simulink model "track5p"  (Simulink 9.0)
settings: Solver=ode1  StartTime=0.0  StopTime=120  RelTol=1e-3
libraries: simulink x2, Solver_SF x1
settings Model: Creator=lancer  LastModifiedBy=lancer
settings DataIOCC: SaveFormat=Dataset
settings OptimizationCC: LifeSpan=auto
settings DebuggingCC: UnderspecifiedInitializationDetection=Simplified  MergeDetectMultiDrivingBlocksExec=error  SFUnexpectedBacktrackingDiag=error  SFNoUnconditionalDefaultTransitionDiag=error  SFExecutionAtInitializationDiag=warning
settings HardwareCC: ProdBitPerPointer=64  ProdBitPerSizeT=64  ProdBitPerPtrDiffT=64  ProdLargestAtomicFloat=Float  ProdIntDivRoundTo=Zero  ProdEndianess=LittleEndian  ProdWordSize=64  ProdHWDeviceType=Intel->x86-64 (Windows64)
settings ModelReferenceCC: PropagateSignalLabelsOutOfModel=on
settings CodeAppCC: StateflowObjectComments=off
settings GRTTargetCC: TargetLangStandard=C99 (ISO)
settings ConfigComp: CovMetricSettings=dwe  CovHtmlReporting=off  CovSaveCumulativeToWorkspaceVar=off  CovSaveSingleToWorkspaceVar=off  CovExternalEMLEnable=on

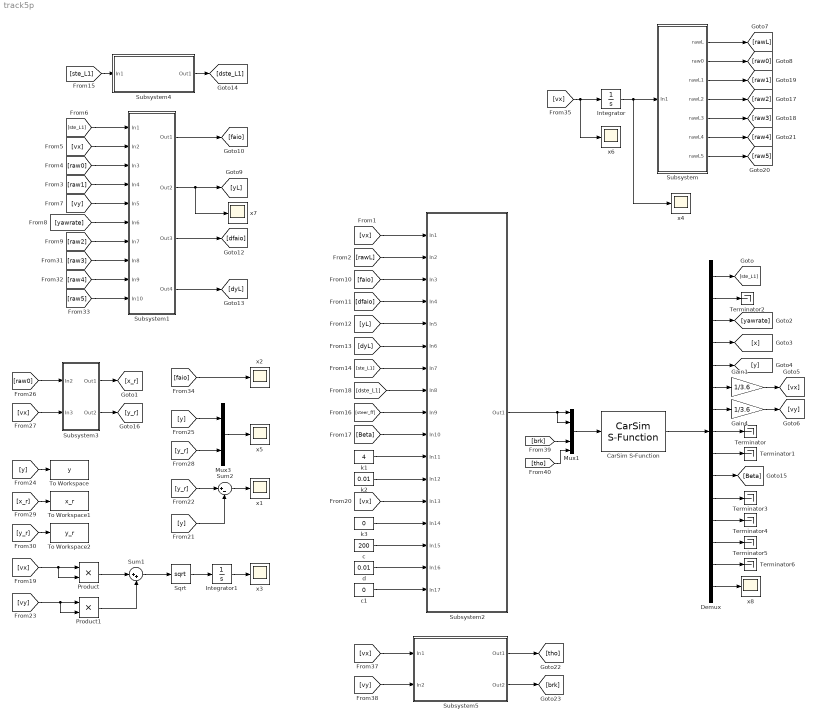
== system track5p ==
  CarSim S-Function : Solver_SF/CarSim S-Function  Priority=1  VehicleCode=i_i  SIMFILE=C:\Users\Public\Documents\CarSim_Data\simfile
  Demux : Demux  Outputs=15
  Gain1 : Gain  Gain=1/3.6
  Gain4 : Gain  Gain=1/3.6
  Integrator : Integrator
  Integrator1 : Integrator
  Mux1 : Mux  Inputs=5
  Mux3 : Mux  Inputs=2
  Product : Product
  Product1 : Product
  Sqrt : Sqrt  SaturateOnIntegerOverflow=on
  Subsystem : Subsystem
  Subsystem1 : Subsystem
  Subsystem2 : Subsystem
  Subsystem3 : Subsystem
  Subsystem4 : Subsystem
  Subsystem5 : Subsystem
  Sum1 : Sum  Inputs=|++
  Sum2 : Sum  Inputs=|+-
  Terminator{,1..6} (7 alike) : Terminator
  To Workspace : ToWorkspace  VariableName=y  SaveFormat=Timeseries  SampleTime=-1
  To Workspace1 : ToWorkspace  VariableName=x_r  SaveFormat=Timeseries  SampleTime=-1
  To Workspace2 : ToWorkspace  VariableName=y_r  SaveFormat=Timeseries  SampleTime=-1
  c : Constant  Value=200
  c1 : Constant  Value=0
  d : Constant  Value=0.01
  k1 : Constant  Value=4
  k2 : Constant  Value=0.01
  k3 : Constant  Value=0
  x{1..8} (8 alike) : Scope
  wires:
  Demux/1 -> [ste_L1]
  Demux/2 -> Terminator2/1
  Demux/3 -> [yawrate]
  Demux/4 -> [x]
  Demux/5 -> [y]
  Demux/8 -> Terminator/1
  Demux/9 -> Terminator1/1
  Demux/10 -> [Beta]
  Demux/11 -> Terminator3/1
  Demux/12 -> Terminator4/1
  Demux/13 -> Terminator5/1
  Demux/14 -> Terminator6/1
  Subsystem/1(rawL) -> [rawL]
  Demux/6 -> Gain1/1
  Gain1/1 -> [vx]
  Gain4/1 -> [vy]
  Demux/7 -> Gain4/1
  [raw0] -> Subsystem3/1(In2)
  [vx] -> Subsystem3/2(In3)
  Subsystem3/1(Out1) -> [x_r]
  Subsystem3/2(Out2) -> [y_r]
  [y_r] -> Sum2/1
  [y] -> Sum2/2
  [y] -> Mux3/1
  [y_r] -> Mux3/2
  Mux3/1 -> x5/1
  Sum2/1 -> x1/1
  [y] -> To Workspace/1
  [x_r] -> To Workspace1/1
  [y_r] -> To Workspace2/1
  Subsystem/2(raw0) -> [raw0]
  Subsystem/3(rawL1) -> [raw1]
  Subsystem/4(rawL2) -> [raw2]
  Subsystem/5(rawL3) -> [raw3]
  Subsystem/6(rawL4) -> [raw4]
  Subsystem/7(rawL5) -> [raw5]
  [faio] -> x2/1
  Mux1/1 -> CarSim S-Function/1
  CarSim S-Function/1 -> Demux/1
  [ste_L1] -> Subsystem1/1(In1)
  [vx] -> Subsystem1/2(In2)
  [raw0] -> Subsystem1/3(In3)
  [raw1] -> Subsystem1/4(In4)
  [vy] -> Subsystem1/5(In5)
  [yawrate] -> Subsystem1/6(In6)
  [raw2] -> Subsystem1/7(In7)
  [raw3] -> Subsystem1/8(In8)
  [raw4] -> Subsystem1/9(In9)
  [raw5] -> Subsystem1/10(In10)
  Subsystem1/1(Out1) -> [faio]
  Subsystem1/2(Out2) -> [yL], x7/1
  Subsystem1/3(Out3) -> [dfaio]
  Subsystem1/4(Out4) -> [dyL]
  Subsystem2/1(Out1) -> Mux1/2, Mux1/1
  [vx] -> Subsystem2/1(In1)
  [rawL] -> Subsystem2/2(In2)
  [faio] -> Subsystem2/3(In3)
  [dfaio] -> Subsystem2/4(In4)
  [yL] -> Subsystem2/5(In5)
  [dyL] -> Subsystem2/6(In6)
  [ste_L1] -> Subsystem2/7(In7)
  [dste_L1] -> Subsystem2/8(In8)
  [steer_ff] -> Subsystem2/9(In9)
  [Beta] -> Subsystem2/10(In10)
  k1/1 -> Subsystem2/11(In11)
  k2/1 -> Subsystem2/12(In12)
  [vx] -> Subsystem2/13(In13)
  k3/1 -> Subsystem2/14(In14)
  c/1 -> Subsystem2/15(In15)
  d/1 -> Subsystem2/16(In16)
  c1/1 -> Subsystem2/17(In17)
  [ste_L1] -> Subsystem4/1(In1)
  Subsystem4/1(Out1) -> [dste_L1]
  [vx] -> Product/2, Product/1
  [vy] -> Product1/2, Product1/1
  Product/1 -> Sum1/1
  Product1/1 -> Sum1/2
  Sum1/1 -> Sqrt/1
  Sqrt/1 -> Integrator1/1
  Integrator1/1 -> x3/1
  [vx] -> x6/1, Integrator/1
  [vx] -> Subsystem5/1(In1)
  [vy] -> Subsystem5/2(In2)
  Subsystem5/2(Out2) -> [brk]
  Subsystem5/1(Out1) -> [tho]
  Integrator/1 -> Subsystem/1(In1), x4/1
  Demux/15 -> x8/1
  [tho] -> Mux1/5
  [brk] -> Mux1/4

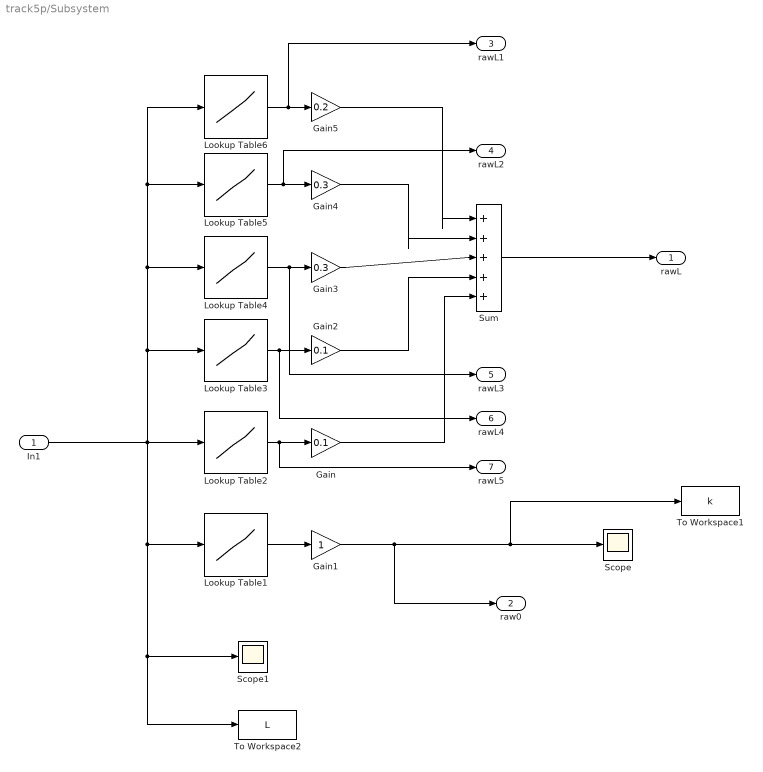
== system track5p/Subsystem ==
  In1 : Inport
  Gain : Gain  Gain=0.1
  Gain1 : Gain
  Gain2 : Gain  Gain=0.1
  Gain3 : Gain  Gain=0.3
  Gain4 : Gain  Gain=0.3
  Gain5 : Gain  Gain=0.2
  Lookup Table1 : Lookup  InputValues=load('change_lane_s.txt')  Table=load('change_lane_p.txt')
  Lookup Table2 : Lookup  InputValues=load('change_lane_s.txt')  Table=load('change_lane_p05.txt')
  Lookup Table3 : Lookup  InputValues=load('change_lane_s.txt')  Table=load('change_lane_p04.txt')
  Lookup Table4 : Lookup  InputValues=load('change_lane_s.txt')  Table=load('change_lane_p03.txt')
  Lookup Table5 : Lookup  InputValues=load('change_lane_s.txt')  Table=load('change_lane_p02.txt')
  Lookup Table6 : Lookup  InputValues=load('change_lane_s.txt')  Table=load('change_lane_p01.txt')
  Scope : Scope
  Scope1 : Scope
  Sum : Sum  Inputs=|+++++
  To Workspace1 : ToWorkspace  VariableName=k  SaveFormat=Timeseries  SampleTime=-1
  To Workspace2 : ToWorkspace  VariableName=L  SaveFormat=Timeseries  SampleTime=-1
  rawL : Outport
  raw0 : Outport  Port=2
  rawL1 : Outport  Port=3
  rawL2 : Outport  Port=4
  rawL3 : Outport  Port=5
  rawL4 : Outport  Port=6
  rawL5 : Outport  Port=7
  wires:
  Gain1/1 -> raw0/1, To Workspace1/1, Scope/1
  Sum/1 -> rawL/1
  Lookup Table1/1 -> Gain1/1
  Lookup Table2/1 -> rawL5/1, Gain/1
  Lookup Table3/1 -> rawL4/1, Gain2/1
  Lookup Table4/1 -> rawL3/1, Gain3/1
  Lookup Table5/1 -> rawL2/1, Gain4/1
  Lookup Table6/1 -> rawL1/1, Gain5/1
  Gain3/1 -> Sum/3
  Gain4/1 -> Sum/2
  Gain5/1 -> Sum/1
  Gain2/1 -> Sum/4
  Gain/1 -> Sum/5
  In1/1 -> Lookup Table3/1, Lookup Table4/1, Lookup Table5/1, Lookup Table6/1, To Workspace2/1, Scope1/1, Lookup Table1/1, Lookup Table2/1

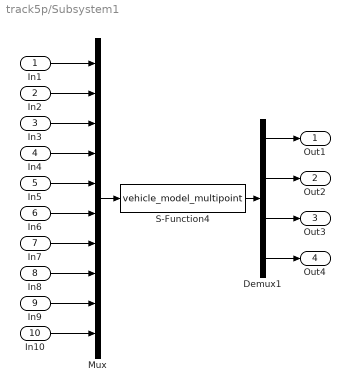
== system track5p/Subsystem1 ==
  In1 : Inport
  In2 : Inport  Port=2
  In3 : Inport  Port=3
  In4 : Inport  Port=4
  In5 : Inport  Port=5
  In6 : Inport  Port=6
  In7 : Inport  Port=7
  In8 : Inport  Port=8
  In9 : Inport  Port=9
  In10 : Inport  Port=10
  Demux1 : Demux
  Mux : Mux  Inputs=10
  S-Function4 : S-Function  FunctionName=vehicle_model_multipoint  SFunctionDeploymentMode=off  EnableBusSupport=off
  Out1 : Outport
  Out2 : Outport  Port=2
  Out3 : Outport  Port=3
  Out4 : Outport  Port=4
  wires:
  Demux1/1 -> Out1/1
  In1/1 -> Mux/1
  Demux1/2 -> Out2/1
  In2/1 -> Mux/2
  S-Function4/1 -> Demux1/1
  Mux/1 -> S-Function4/1
  In4/1 -> Mux/4
  In3/1 -> Mux/3
  In5/1 -> Mux/5
  In6/1 -> Mux/6
  Demux1/3 -> Out3/1
  Demux1/4 -> Out4/1
  In9/1 -> Mux/9
  In8/1 -> Mux/8
  In7/1 -> Mux/7
  In10/1 -> Mux/10

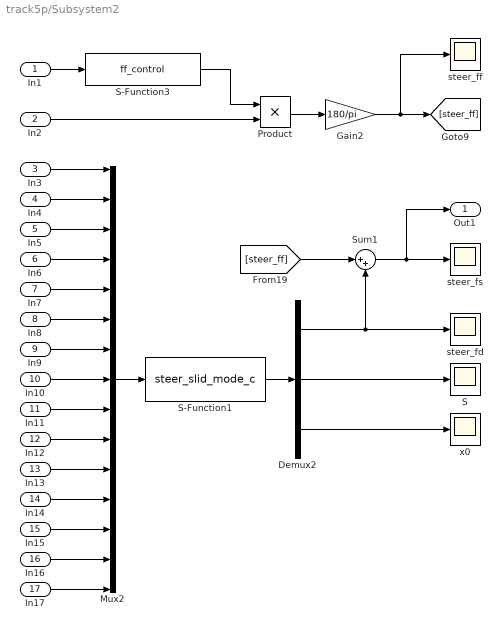
== system track5p/Subsystem2 ==
  In1 : Inport
  In2 : Inport  Port=2
  In3 : Inport  Port=3
  In4 : Inport  Port=4
  In5 : Inport  Port=5
  In6 : Inport  Port=6
  In7 : Inport  Port=7
  In8 : Inport  Port=8
  In9 : Inport  Port=9
  In10 : Inport  Port=10
  In11 : Inport  Port=11
  In12 : Inport  Port=12
  In13 : Inport  Port=13
  In14 : Inport  Port=14
  In15 : Inport  Port=15
  In16 : Inport  Port=16
  In17 : Inport  Port=17
  Demux2 : Demux  Outputs=3
  Gain2 : Gain  Gain=180/pi
  Mux2 : Mux  Inputs=15
  Product : Product
  S : Scope
  S-Function1 : S-Function  FunctionName=steer_slid_mode_c  SFunctionDeploymentMode=off  EnableBusSupport=off
  S-Function3 : S-Function  FunctionName=ff_control  SFunctionDeploymentMode=off  EnableBusSupport=off
  Sum1 : Sum  Inputs=|++
  steer_fd : Scope
  steer_ff : Scope
  steer_fs : Scope
  x0 : Scope
  Out1 : Outport
  wires:
  In1/1 -> S-Function3/1
  In2/1 -> Product/2
  S-Function3/1 -> Product/1
  In16/1 -> Mux2/14
  Sum1/1 -> Out1/1, steer_fs/1
  In7/1 -> Mux2/5
  In17/1 -> Mux2/15
  Gain2/1 -> steer_ff/1, [steer_ff]
  Demux2/2 -> S/1
  In3/1 -> Mux2/1
  In12/1 -> Mux2/10
  In11/1 -> Mux2/9
  In13/1 -> Mux2/11
  In15/1 -> Mux2/13
  In6/1 -> Mux2/4
  In14/1 -> Mux2/12
  Product/1 -> Gain2/1
  In9/1 -> Mux2/7
  Demux2/3 -> x0/1
  In5/1 -> Mux2/3
  Demux2/1 -> Sum1/2, steer_fd/1
  In4/1 -> Mux2/2
  In10/1 -> Mux2/8
  In8/1 -> Mux2/6
  S-Function1/1 -> Demux2/1
  Mux2/1 -> S-Function1/1
  [steer_ff] -> Sum1/1

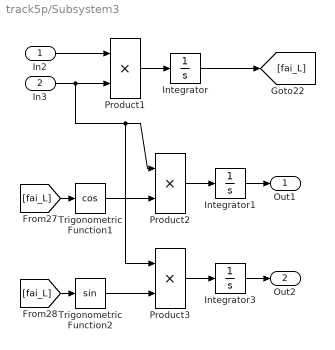
== system track5p/Subsystem3 ==
  In2 : Inport
  In3 : Inport  Port=2
  Integrator : Integrator
  Integrator1 : Integrator
  Integrator3 : Integrator
  Product1 : Product  RndMeth=Zero
  Product2 : Product  RndMeth=Zero
  Product3 : Product  RndMeth=Zero
  Trigonometric Function1 : Trigonometry  Operator=cos
  Trigonometric Function2 : Trigonometry
  Out1 : Outport
  Out2 : Outport  Port=2
  wires:
  In3/1 -> Product3/1, Product2/1, Product1/2
  Product1/1 -> Integrator/1
  [fai_L] -> Trigonometric Function1/1
  Trigonometric Function1/1 -> Product2/2
  Product2/1 -> Integrator1/1
  [fai_L] -> Trigonometric Function2/1
  Trigonometric Function2/1 -> Product3/2
  Product3/1 -> Integrator3/1
  Integrator/1 -> [fai_L]
  In2/1 -> Product1/1
  Integrator1/1 -> Out1/1
  Integrator3/1 -> Out2/1

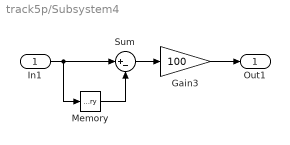
== system track5p/Subsystem4 ==
  In1 : Inport
  Gain3 : Gain  Gain=100
  Memory : Memory
  Sum : Sum  Inputs=|+-
  Out1 : Outport
  wires:
  In1/1 -> Memory/1, Sum/1
  Memory/1 -> Sum/2
  Sum/1 -> Gain3/1
  Gain3/1 -> Out1/1

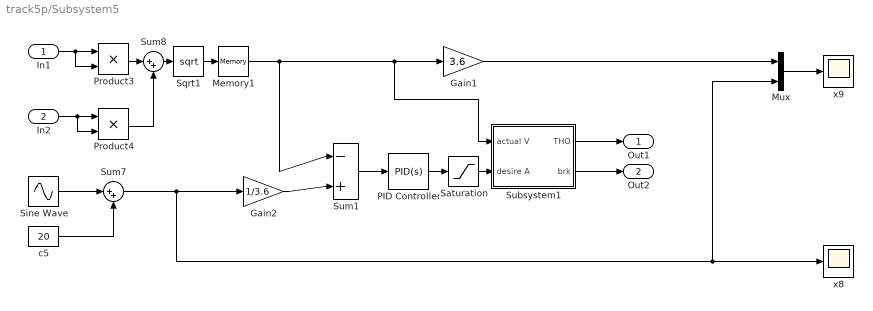
== system track5p/Subsystem5 ==
  In1 : Inport
  In2 : Inport  Port=2
  Gain1 : Gain  Gain=3.6
  Gain2 : Gain  Gain=1/3.6
  Memory1 : Memory
  Mux : Mux  Inputs=2
  PID Controller : simulink/Continuous/PID Controller  Controller=PID  TimeDomain=Continuous-time  SampleTime=-1  IntegratorMethod=Forward Euler  FilterMethod=Forward Euler  Form=Parallel  UseFilter=on  ControllerParametersSource=internal  P=8  I=1  D=0.05  N=100  InitialConditionSource=internal  InitialConditionForIntegrator=0  InitialConditionForFilter=0  ExternalReset=none  LimitOutput=off  UpperSaturationLimit=inf  LowerSaturationLimit=-inf  LinearizeAsGain=on  AntiWindupMode=none  Kb=1  TrackingMode=off  Kt=1  PParamMin=[]  PParamMax=[]  IParamMin=[]  IParamMax=[]  DParamMin=[]  DParamMax=[]  NParamMin=[]  NParamMax=[]  KbParamMin=[]  KbParamMax=[]  KtParamMin=[]  KtParamMax=[]  POutMin=[]  POutMax=[]  IOutMin=[]  IOutMax=[]  DOutMin=[]  DOutMax=[]  NOutMin=[]  NOutMax=[]  KbOutMin=[]  KbOutMax=[]  KtOutMin=[]  KtOutMax=[]  IntegratorOutMin=[]  IntegratorOutMax=[]  FilterOutMin=[]  FilterOutMax=[]  SumOutMin=[]  SumOutMax=[]  SumI1OutMin=[]  SumI1OutMax=[]  SumI2OutMin=[]  SumI2OutMax=[]  SumI3OutMin=[]  SumI3OutMax=[]  SumDOutMin=[]  SumDOutMax=[]  SaturationOutMin=[]  SaturationOutMax=[]  IntegratorContinuousStateAttributes=''  IntegratorStateMustResolveToSignalObject=off  IntegratorRTWStateStorageClass=Auto  FilterContinuousStateAttributes=''  FilterStateMustResolveToSignalObject=off  FilterRTWStateStorageClass=Auto  DifferentiatorICPrevScaledInput=0  DifferentiatorOutMin=[]  DifferentiatorOutMax=[]  InitialConditionSetting=State (most efficient)  FilterDiffOutCoefMin=[]  FilterDiffOutCoefMax=[]  SumDenOutMin=[]  SumDenOutMax=[]  SumNumOutMin=[]  SumNumOutMax=[]  ReciprocalOutMin=[]  ReciprocalOutMax=[]  DivideOutMin=[]  DivideOutMax=[]  TunerSelectOption=Transfer Function Based (PID Tuner App)
  Product3 : Product
  Product4 : Product
  Saturation : Saturate  UpperLimit=3  LowerLimit=-3
  Sine Wave : Sin  Amplitude=5  Frequency=0.1  SampleTime=0
  Sqrt1 : Sqrt  SaturateOnIntegerOverflow=on
  Subsystem1 : Subsystem
  Sum1 : Sum  Inputs=|-+
  Sum7 : Sum  Inputs=|++
  Sum8 : Sum  Inputs=|++
  c5 : Constant  Value=20
  x8 : Scope
  x9 : Scope
  Out1 : Outport
  Out2 : Outport  Port=2
  wires:
  Sine Wave/1 -> Sum7/1
  Subsystem1/1(THO) -> Out1/1
  Sqrt1/1 -> Memory1/1
  Sum8/1 -> Sqrt1/1
  Subsystem1/2(brk) -> Out2/1
  In2/1 -> Product4/2, Product4/1
  Product4/1 -> Sum8/2
  Product3/1 -> Sum8/1
  In1/1 -> Product3/2, Product3/1
  Memory1/1 -> Subsystem1/1(actual V), Gain1/1, Sum1/1
  PID Controller/1 -> Saturation/1
  Saturation/1 -> Subsystem1/2(desire A)
  c5/1 -> Sum7/2
  Sum1/1 -> PID Controller/1
  Sum7/1 -> Mux/2, x8/1, Gain2/1
  Gain1/1 -> Mux/1
  Mux/1 -> x9/1
  Gain2/1 -> Sum1/2

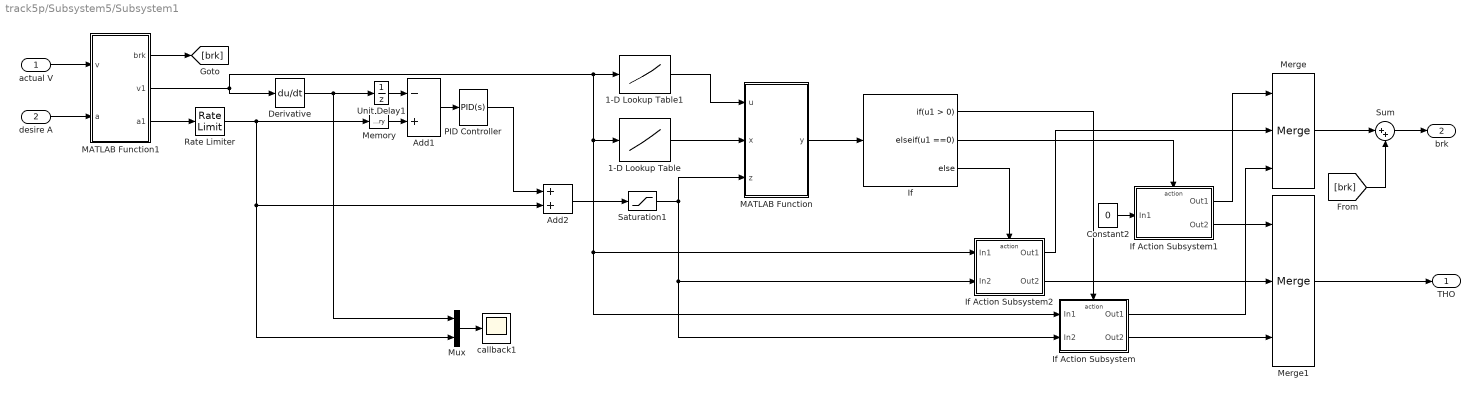
== system track5p/Subsystem5/Subsystem1 ==
  actual V : Inport
  desire A : Inport  Port=2
  1-D Lookup Table : Lookup_n-D  NumberOfTableDimensions=1  BreakpointsForDimension1=xlsread('tho0brk0','sheet4','A2:A16')  Table=xlsread('tho0brk0','sheet4','B2:B16')  InternalRulePriority=Speed  RndMeth=Simplest  InputSameDT=on
  1-D Lookup Table1 : Lookup_n-D  NumberOfTableDimensions=1  BreakpointsForDimension1=xlsread('tho0brk0','sheet3','A2:A29')  Table=xlsread('tho0brk0','sheet3','B2:B29')  InternalRulePriority=Speed  RndMeth=Simplest  InputSameDT=on
  Add1 : Sum  Inputs=-+
  Add2 : Sum
  Constant2 : Constant  Value=0
  Derivative : Derivative
  If : If  ElseIfExpressions=u1 ==0
  If Action Subsystem : Subsystem  TreatAsAtomicUnit=on
  If Action Subsystem1 : Subsystem  TreatAsAtomicUnit=on
  If Action Subsystem2 : Subsystem  TreatAsAtomicUnit=on
  MATLAB Function : MATLAB Function  TreatAsAtomicUnit=on
  MATLAB Function1 : MATLAB Function  TreatAsAtomicUnit=on
  Memory : Memory
  Merge : Merge  Inputs=3
  Merge1 : Merge  Inputs=3
  Mux : Mux  Inputs=2
  PID Controller : simulink/Continuous/PID Controller  Controller=PID  TimeDomain=Continuous-time  SampleTime=-1  IntegratorMethod=Forward Euler  FilterMethod=Forward Euler  Form=Parallel  UseFilter=on  ControllerParametersSource=internal  P=2  I=4  D=0.005  N=100  InitialConditionSource=internal  InitialConditionForIntegrator=0  InitialConditionForFilter=0  ExternalReset=none  LimitOutput=off  UpperSaturationLimit=inf  LowerSaturationLimit=-inf  LinearizeAsGain=on  AntiWindupMode=none  Kb=1  TrackingMode=off  Kt=1  PParamMin=[]  PParamMax=[]  IParamMin=[]  IParamMax=[]  DParamMin=[]  DParamMax=[]  NParamMin=[]  NParamMax=[]  KbParamMin=[]  KbParamMax=[]  KtParamMin=[]  KtParamMax=[]  POutMin=[]  POutMax=[]  IOutMin=[]  IOutMax=[]  DOutMin=[]  DOutMax=[]  NOutMin=[]  NOutMax=[]  KbOutMin=[]  KbOutMax=[]  KtOutMin=[]  KtOutMax=[]  IntegratorOutMin=[]  IntegratorOutMax=[]  FilterOutMin=[]  FilterOutMax=[]  SumOutMin=[]  SumOutMax=[]  SumI1OutMin=[]  SumI1OutMax=[]  SumI2OutMin=[]  SumI2OutMax=[]  SumI3OutMin=[]  SumI3OutMax=[]  SumDOutMin=[]  SumDOutMax=[]  SaturationOutMin=[]  SaturationOutMax=[]  IntegratorContinuousStateAttributes=''  IntegratorStateMustResolveToSignalObject=off  IntegratorRTWStateStorageClass=Auto  FilterContinuousStateAttributes=''  FilterStateMustResolveToSignalObject=off  FilterRTWStateStorageClass=Auto  DifferentiatorICPrevScaledInput=0  DifferentiatorOutMin=[]  DifferentiatorOutMax=[]  InitialConditionSetting=State (most efficient)  FilterDiffOutCoefMin=[]  FilterDiffOutCoefMax=[]  SumDenOutMin=[]  SumDenOutMax=[]  SumNumOutMin=[]  SumNumOutMax=[]  ReciprocalOutMin=[]  ReciprocalOutMax=[]  DivideOutMin=[]  DivideOutMax=[]  TunerSelectOption=Transfer Function Based (PID Tuner App)
  Rate Limiter : RateLimiter  RisingSlewLimit=15  FallingSlewLimit=-20  SampleTimeMode=inherited
  Saturation1 : Saturate  UpperLimit=5.4  LowerLimit=-5
  Sum : Sum  Inputs=|++
  Unit Delay1 : UnitDelay  SampleTime=-1
  callback1 : Scope
  THO : Outport
  brk : Outport  Port=2
  wires:
  If Action Subsystem2/1(Out1) -> Merge/2
  Saturation1/1 -> If Action Subsystem/2(In2), If Action Subsystem2/2(In2), MATLAB Function/3(z)
  Merge1/1 -> THO/1
  If Action Subsystem/2(Out2) -> Merge1/3
  If Action Subsystem1/1(Out1) -> Merge/1
  If/2 -> If Action Subsystem1/Action
  Add1/1 -> PID Controller/1
  If/1 -> If Action Subsystem/Action
  If Action Subsystem/1(Out1) -> Merge/3
  If/3 -> If Action Subsystem2/Action
  Add2/1 -> Saturation1/1
  Memory/1 -> Add1/2
  Constant2/1 -> If Action Subsystem1/1(In1)
  If Action Subsystem2/2(Out2) -> Merge1/2
  1-D Lookup Table/1 -> MATLAB Function/2(x)
  Unit Delay1/1 -> Add1/1
  Merge/1 -> Sum/1
  If Action Subsystem1/2(Out2) -> Merge1/1
  PID Controller/1 -> Add2/1
  1-D Lookup Table1/1 -> MATLAB Function/1(u)
  MATLAB Function/1(y) -> If/1
  Derivative/1 -> Unit Delay1/1, Mux/1
  Mux/1 -> callback1/1
  MATLAB Function1/2(v1) -> 1-D Lookup Table/1, If Action Subsystem2/1(In1), If Action Subsystem/1(In1), 1-D Lookup Table1/1, Derivative/1
  actual V/1 -> MATLAB Function1/1(v)
  desire A/1 -> MATLAB Function1/2(a)
  MATLAB Function1/1(brk) -> [brk]
  Sum/1 -> brk/1
  [brk] -> Sum/2
  MATLAB Function1/3(a1) -> Rate Limiter/1
  Rate Limiter/1 -> Mux/2, Add2/2, Memory/1

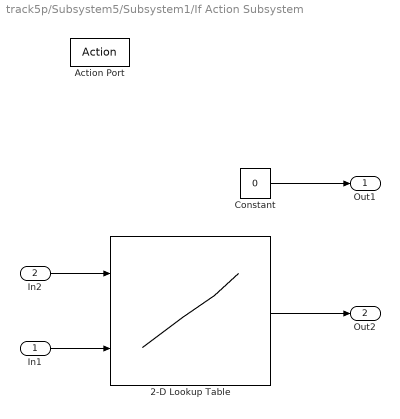
== system track5p/Subsystem5/Subsystem1/If Action Subsystem ==
  In1 : Inport
  In2 : Inport  Port=2
  Action Port : ActionPort  ActionType=then
  2-D Lookup Table : Lookup_n-D  BreakpointsForDimension1=xlsread('tho-v-a','sheet4','A3:A38')  BreakpointsForDimension2=xlsread('tho-v-a','sheet4','B2:P2')  Table=xlsread('tho-v-a','sheet4','B3:P38')  InternalRulePriority=Speed  RndMeth=Simplest  InputSameDT=on
  Constant : Constant  Value=0
  Out1 : Outport
  Out2 : Outport  Port=2
  wires:
  Constant/1 -> Out1/1
  2-D Lookup Table/1 -> Out2/1
  In2/1 -> 2-D Lookup Table/1
  In1/1 -> 2-D Lookup Table/2

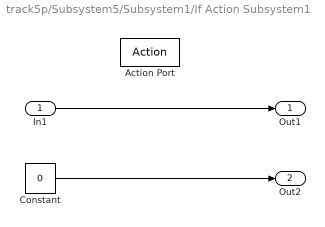
== system track5p/Subsystem5/Subsystem1/If Action Subsystem1 ==
  In1 : Inport
  Action Port : ActionPort  ActionType=elseif
  Constant : Constant  Value=0
  Out1 : Outport
  Out2 : Outport  Port=2
  wires:
  In1/1 -> Out1/1
  Constant/1 -> Out2/1

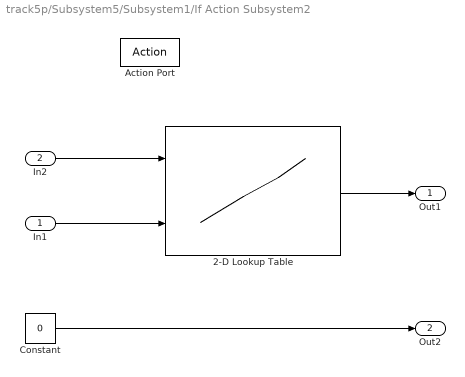
== system track5p/Subsystem5/Subsystem1/If Action Subsystem2 ==
  In1 : Inport
  In2 : Inport  Port=2
  Action Port : ActionPort  ActionType=else
  2-D Lookup Table : Lookup_n-D  BreakpointsForDimension1=xlsread('brk-v-a','sheet3','A3:A28')  BreakpointsForDimension2=xlsread('brk-v-a','sheet3','B2:P2')  Table=xlsread('brk-v-a','sheet3','B3:P28')  InternalRulePriority=Speed  RndMeth=Simplest  InputSameDT=on
  Constant : Constant  Value=0
  Out1 : Outport
  Out2 : Outport  Port=2
  wires:
  2-D Lookup Table/1 -> Out1/1
  Constant/1 -> Out2/1
  In2/1 -> 2-D Lookup Table/1
  In1/1 -> 2-D Lookup Table/2

== matlab function Subsystem5/Subsystem1/MATLAB Function ==
  data: u input double; y output double; x input double; z input double
function y = fcn(u, x, z)
if z>u
    y=1;
elseif z<u&&z>x
    y=0;
elseif z<x
    y=-1;
else
    y=5;
end

== matlab function Subsystem5/Subsystem1/MATLAB Function1 ==
  data: v input double; brk output double; v1 output double; a1 output double; a input double
function [brk, v1, a1] = fcn(v, a)
if v<=0.4&&a<=-3
    brk=2*v+0.7;
    v1=v;
    a1=0;
else
    v1=v;
    a1=a;
    brk=0;
end
